simulink model "inverter_120degree"  (Simulink 7.3)
settings: Solver=ode23tb  StartTime=0.0  StopTime=0.1  MaxStep=1e-5  RelTol=1e-3
libraries: powerlib x20, simulink x1
settings Model: Creator=viswam  LastModifiedBy=viswam
settings SolverCC: InitialStep=1e-6
settings OptimizationCC: InitFltsAndDblsToZero=on
settings DebuggingCC: SaveWithParameterizedLinksMsg=none  SignalResolutionControl=TryResolveAllWithWarning  MultiTaskDSMMsg=warning  MultiTaskCondExecSysMsg=none
settings RTWCC: IncludeERTFirstTime=on
settings GRTTargetCC: TargetFcnLib=ansi_tfl_tmw.mat

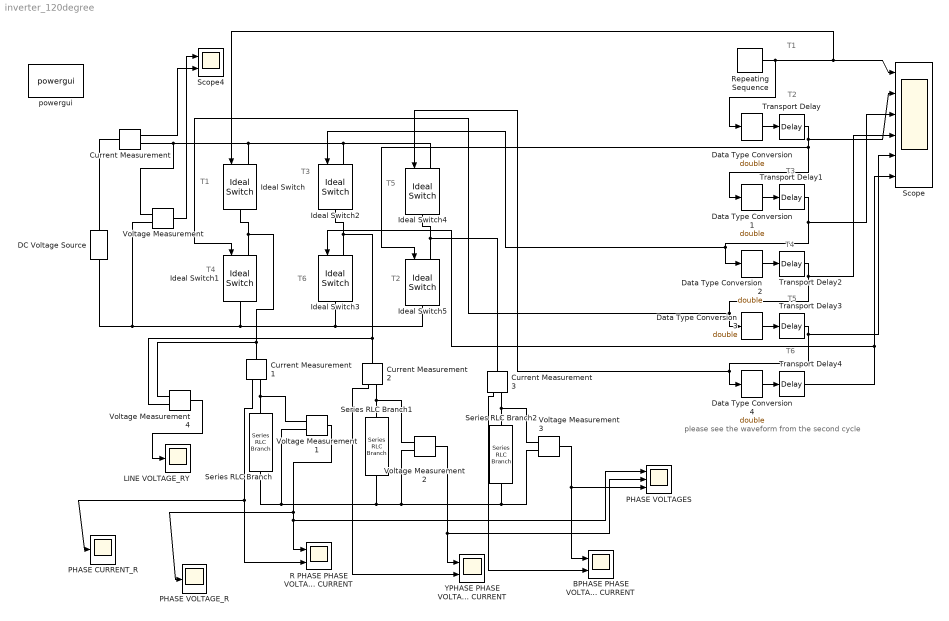
== system inverter_120degree ==
  note: T1
  note: T2
  note: T3
  note: T4
  note: T5
  note: T6
  note: T1
  note: T2
  note: T3
  note: T4
  note: T5
  note: T6
  note: please see the waveform from the second cycle
  BPHASE PHASE VOLTAGE & CURRENT : Scope  NumInputPorts=2
      settings: TimeRange=0.04  YMin=-5~-5  YMax=5~5  SaveName=ScopeData3
  Current Measurement{,1..3} (4 alike) : powerlib/Measurements/Current Measurement  DialogController=POWERSYS.PowerSysDialog  SystemSampleTime=-1  PhasorSimulation=off  OutputType=Complex  PSBequivalent=0
  DC Voltage Source : powerlib/Electrical Sources/DC Voltage Source  DialogController=POWERSYS.PowerSysDialog  SystemSampleTime=-1  Amplitude=300  Measurements=None
  Data Type Conversion{,1..4} (5 alike) : DataTypeConversion  OutDataTypeMode=double  OutDataType=sfix(16)  OutScaling=2^0  OutDataTypeStr=double
  Ideal Switch{,1..5} (6 alike) : powerlib/Power Electronics/Ideal Switch  DialogController=POWERSYS.PowerSysDialog  SystemSampleTime=-1  Ron=0.001  Lon=0  IC=0  Rs=1e5  Cs=inf  Measurements=off
  LINE VOLTAGE_RY : Scope
      settings: TimeRange=0.04  SaveName=RYVOLTAGES  SampleInput=on  SampleTime=1e-6
  PHASE CURRENT_R : Scope
      settings: TimeRange=0.04  SaveName=PHASECURRENT_R  SampleInput=on  SampleTime=1e-6
  PHASE VOLTAGES : Scope  NumInputPorts=3
      settings: TimeRange=0.06  YMin=-200~0~-150  YMax=25~200~150  SaveName=ScopeData5
  PHASE VOLTAGE_R : Scope
      settings: TimeRange=0.04  SaveName=PHASEVOLTAGE_R  SampleInput=on  SampleTime=1e-6
  R PHASE PHASE VOLTAGE & CURRENT : Scope  NumInputPorts=2
      settings: TimeRange=0.04  YMin=-5~-5  YMax=5~5
  Repeating Sequence : simulink/Sources/Repeating Sequence  SystemSampleTime=-1  rep_seq_t=[0 0 6.667e-3 6.667e-3 10e-3 20e-3]  rep_seq_y=[0 1 1 0 0 0]
  Scope : Scope  NumInputPorts=6
      settings: TimeRange=0.02  YMin=-5~-5~-5~-5~-5~-5  YMax=5~5~5~5~5~5
  Scope4 : Scope  NumInputPorts=2
      settings: TimeRange=0.04  YMin=-5~-5  YMax=5~5  SaveName=ScopeData4
  Series RLC Branch : powerlib/Elements/Series RLC Branch  DialogController=POWERSYS.PowerSysDialog  PhysicalDomain=powersysdomain  SubClassName=unknown  LeftPortType=p1  RightPortType=p1  LConnTagsString=__new0  RConnTagsString=__new0  BranchType=R  Resistance=10  Inductance=1e-3  SetiL0=off  InitialCurrent=0  Capacitance=1e-6  Setx0=off  InitialVoltage=0  Measurements=None
  Series RLC Branch1 : powerlib/Elements/Series RLC Branch  DialogController=POWERSYS.PowerSysDialog  PhysicalDomain=powersysdomain  SubClassName=unknown  LeftPortType=p1  RightPortType=p1  LConnTagsString=__new0  RConnTagsString=__new0  BranchType=R  Resistance=10  Inductance=1e-3  SetiL0=off  InitialCurrent=0  Capacitance=1e-6  Setx0=off  InitialVoltage=0  Measurements=None
  Series RLC Branch2 : powerlib/Elements/Series RLC Branch  DialogController=POWERSYS.PowerSysDialog  PhysicalDomain=powersysdomain  SubClassName=unknown  LeftPortType=p1  RightPortType=p1  LConnTagsString=__new0  RConnTagsString=__new0  BranchType=R  Resistance=10  Inductance=1e-3  SetiL0=off  InitialCurrent=0  Capacitance=1e-6  Setx0=off  InitialVoltage=0  Measurements=None
  Transport Delay{,1..4} (5 alike) : TransportDelay  DelayTime=3.33e-3
  Voltage Measurement{,1..4} (5 alike) : powerlib/Measurements/Voltage Measurement  DialogController=POWERSYS.PowerSysDialog  SystemSampleTime=-1  PhasorSimulation=off  OutputType=Complex  PSBequivalent=0
  YPHASE PHASE VOLTAGE & CURRENT : Scope  NumInputPorts=2
      settings: TimeRange=0.04  YMin=-5~-5  YMax=5~5  SaveName=ScopeData2
  powergui : powerlib/powergui  Priority=1  SystemSampleTime=-1  SimulationMode=Continuous  SampleTime=50e-6  frequency=60  SPID=off  DisableSnubberDevices=off  DisableRonSwitches=off  DisableVfSwitches=off  SwTol=0  Interpol=off  frequencyindice=0  echomessages=off  HookPort=off  DisplayEquations=off  FunctionMessages=off  EnableUseOfTLC=off  x0status=blocks  RestoreLinks=warning  Frange=[0:2:500]  Ylog=off  Xlog=on  ShowGrid=off  save=off  variable=ZData  ZoomFFT=on  StartTime=0.0  cycles=1  DisplayStyle=1  fundamental=60  FreqAxis=off  MaxFrequency=1000  frequencyindicesteady=1  RmsSteady=1  display=off  Ts=0  methode=off
  wires:
  Data Type Conversion/1 -> Transport Delay/1
  Repeating Sequence/1 -> Data Type Conversion/1, Scope/1, Ideal Switch/1
  Transport Delay/1 -> Scope/2, Data Type Conversion1/1, Ideal Switch5/1
  Transport Delay1/1 -> Scope/3, Data Type Conversion2/1, Ideal Switch2/1
  Transport Delay2/1 -> Scope/4, Data Type Conversion3/1, Ideal Switch1/1
  Transport Delay3/1 -> Scope/5, Data Type Conversion4/1, Ideal Switch4/1
  Data Type Conversion1/1 -> Transport Delay1/1
  Data Type Conversion2/1 -> Transport Delay2/1
  Data Type Conversion3/1 -> Transport Delay3/1
  Data Type Conversion4/1 -> Transport Delay4/1
  Transport Delay4/1 -> Scope/6, Ideal Switch3/1
  Voltage Measurement1/1 -> R PHASE PHASE VOLTAGE & CURRENT/1, PHASE VOLTAGES/1, PHASE VOLTAGE_R/1
  Current Measurement1/1 -> R PHASE PHASE VOLTAGE & CURRENT/2, PHASE CURRENT_R/1
  Voltage Measurement2/1 -> PHASE VOLTAGES/2, YPHASE PHASE VOLTAGE & CURRENT/1
  Current Measurement2/1 -> YPHASE PHASE VOLTAGE & CURRENT/2
  Voltage Measurement3/1 -> PHASE VOLTAGES/3, BPHASE PHASE VOLTAGE & CURRENT/1
  Current Measurement3/1 -> BPHASE PHASE VOLTAGE & CURRENT/2
  Voltage Measurement/1 -> Scope4/1
  Current Measurement/1 -> Scope4/2
  Voltage Measurement4/1 -> LINE VOLTAGE_RY/1
  connections:
  Ideal Switch/RConn1 -- Ideal Switch1/LConn1 -- Current Measurement1/LConn1 -- Voltage Measurement4/LConn1
  Ideal Switch2/RConn1 -- Ideal Switch3/LConn1 -- Current Measurement2/LConn1 -- Voltage Measurement4/LConn2
  Ideal Switch4/RConn1 -- Ideal Switch5/LConn1 -- Current Measurement3/LConn1
  Current Measurement/RConn1 -- Ideal Switch/LConn1 -- Ideal Switch4/LConn1 -- Ideal Switch2/LConn1 -- Voltage Measurement/LConn1
  Ideal Switch1/RConn1 -- Ideal Switch5/RConn1 -- Ideal Switch3/RConn1 -- DC Voltage Source/LConn1 -- Voltage Measurement/LConn2
  DC Voltage Source/RConn1 -- Current Measurement/LConn1
  Series RLC Branch/LConn1 -- Current Measurement1/RConn1 -- Voltage Measurement1/LConn1
  Series RLC Branch1/LConn1 -- Current Measurement2/RConn1 -- Voltage Measurement2/LConn1
  Series RLC Branch2/LConn1 -- Current Measurement3/RConn1 -- Voltage Measurement3/LConn1
  Series RLC Branch1/RConn1 -- Series RLC Branch/RConn1 -- Voltage Measurement1/LConn2 -- Voltage Measurement2/LConn2 -- Series RLC Branch2/RConn1 -- Voltage Measurement3/LConn2
